simulink model "phasor08_ieee13_2_sc_console"  (Simulink 10.2)
settings: Solver=ode4  StartTime=0.0  StopTime=inf  FixedStep=0.01  RelTol=1e-3
PreLoadFcn:
  | Ts=0.01;
PostLoadFcn:
  | Ts=0.01;
InitFcn:
  | Ts=0.01;
StartFcn:
  | Ts=0.01;
libraries: opal_lib x2
settings Model: Creator=ZhiqiZhao  LastModifiedBy=xjk374
settings DataIOCC: LimitDataPoints=on
settings OptimizationCC: ExpressionDepthLimit=2147483647  LocalBlockOutputs=off
settings DebuggingCC: SolverPrmCheckMsg=warning  AllowSymbolicDim=off  StateNameClashWarn=warning
settings RTWCC: GenCodeOnly=on

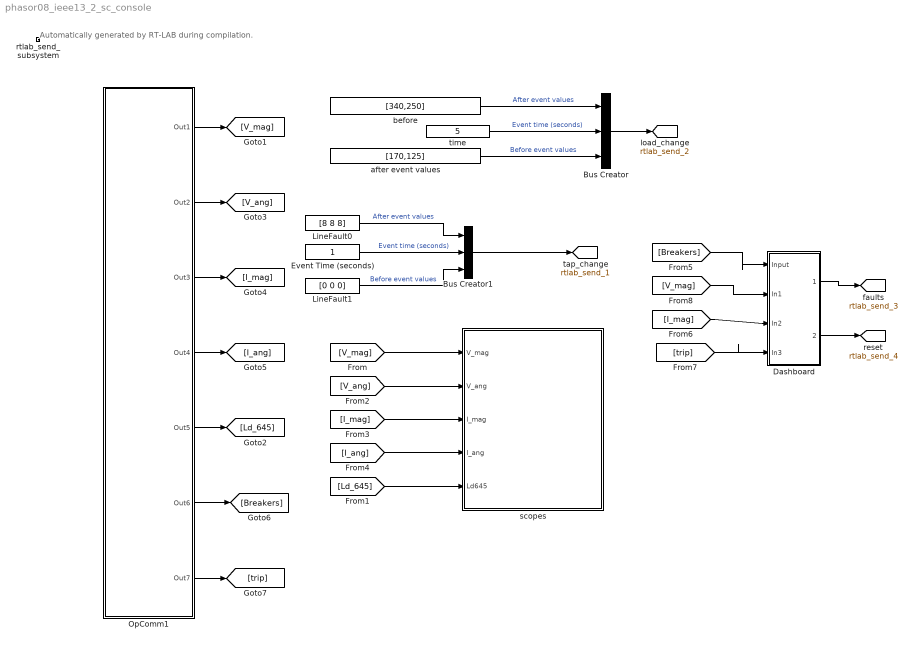
== system phasor08_ieee13_2_sc_console ==
  note: Automatically generated by RT-LAB during compilation.
  Bus Creator : BusCreator  Inputs=3
  Bus Creator1 : BusCreator  Inputs=3
  Dashboard : Subsystem
  Event Time (seconds) : Constant
  LineFault0 : Constant  Value=[8 8 8]
  LineFault1 : Constant  Value=[0 0 0]
  OpComm1 : Subsystem
      mask init:
      | opmaskdisplay('maskdisplay_block',gcb,'disp(''OpComm'')');
      mask Display:
      | patch([0 0.5 0.7 0],[1 1 0 0],[0.7 0.75 0.9]);
      | patch([1 0.53 0.73 1],[1 1 0 0],[1 0.8 0.7]);
      | plot([0 0 1 1 0],[0 1 1 0 0]);
      | disp('OpComm')
  after event values : Constant  Value=[170,125]
  before : Constant  Value=[340,250]
  rtlab_send_subsystem : Subsystem  Priority=-100
      mask Display: text(0,0,'');
  scopes : Subsystem
  time : Constant  Value=5
  tag scope: rtlab_send_1=global, rtlab_send_2=global, rtlab_send_3=global, rtlab_send_4=global
  wires:
  [V_mag] -> Dashboard/2(In1)
  Dashboard/2(Output1) -> [rtlab_send_4]
  [trip] -> Dashboard/4(In3)
  OpComm1/7(Out7) -> [trip]
  [I_mag] -> Dashboard/3(In2)
  Dashboard/1(Output) -> [rtlab_send_3]
  [Breakers] -> Dashboard/1(Input)
  OpComm1/6(Out6) -> [Breakers]
  [Ld_645] -> scopes/5(Ld645)
  [I_ang] -> scopes/4(I_ang)
  [I_mag] -> scopes/3(I_mag)
  [V_ang] -> scopes/2(V_ang)
  [V_mag] -> scopes/1(V_mag)
  OpComm1/3(Out3) -> [I_mag]
  OpComm1/4(Out4) -> [I_ang]
  OpComm1/5(Out5) -> [Ld_645]
  after event values/1 -> Bus Creator/3  "Before event values"
  before/1 -> Bus Creator/1  "After event values"
  Bus Creator1/1 -> [rtlab_send_1]
  Event Time (seconds)/1 -> Bus Creator1/2  "Event time (seconds)"
  LineFault1/1 -> Bus Creator1/3  "Before event values"
  LineFault0/1 -> Bus Creator1/1  "After event values"
  Bus Creator/1 -> [rtlab_send_2]
  time/1 -> Bus Creator/2  "Event time (seconds)"
  OpComm1/2(Out2) -> [V_ang]
  OpComm1/1(Out1) -> [V_mag]

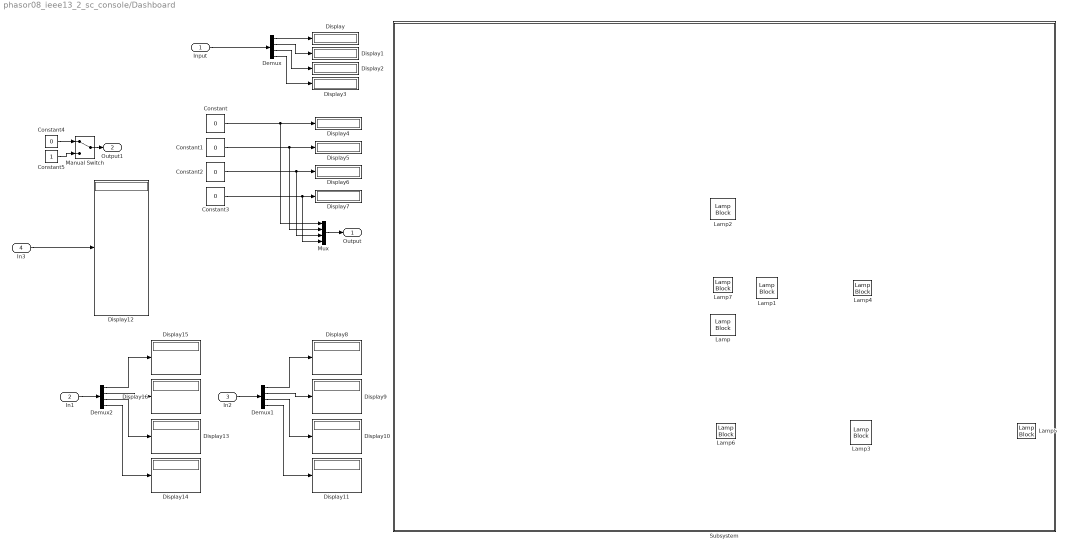
== system phasor08_ieee13_2_sc_console/Dashboard ==
  Input : Inport
  In1 : Inport  Port=2
  In2 : Inport  Port=3
  In3 : Inport  Port=4
  Constant{,1..4} (5 alike) : Constant  Value=0
  Constant5 : Constant
  Demux : Demux
  Demux1 : Demux
  Demux2 : Demux
  Display{,1..16} (17 alike) : Display
  Lamp : LampBlock  LabelPosition=Hide  DefaultColor=DataTag1  States=DataTag2
  Lamp1 : LampBlock  LabelPosition=Hide  DefaultColor=DataTag4  States=DataTag5
  Lamp2 : LampBlock  LabelPosition=Hide  DefaultColor=DataTag7  States=DataTag8
  Lamp3 : LampBlock  LabelPosition=Hide  DefaultColor=DataTag10  States=DataTag11
  Lamp4 : LampBlock  LabelPosition=Hide  DefaultColor=DataTag13  States=DataTag14
  Lamp5 : LampBlock  LabelPosition=Hide  DefaultColor=DataTag16  States=DataTag17
  Lamp6 : LampBlock  LabelPosition=Hide  DefaultColor=DataTag19  States=DataTag20
  Lamp7 : LampBlock  LabelPosition=Hide  DefaultColor=DataTag22  States=DataTag23
  Manual Switch : ManualSwitch
  Mux : Mux
  Subsystem : Subsystem
      mask Display: image('C:\Users\xjk374\OneDrive\0x_Adaptive_Protection\ieee13 with relays.png'); % Use "Edit Image" on toolstrip to change.
  Output : Outport
  Output1 : Outport  Port=2
  wires:
  Demux/1 -> Display/1
  Demux/2 -> Display1/1
  Demux/3 -> Display2/1
  Demux/4 -> Display3/1
  Input/1 -> Demux/1
  Constant/1 -> Mux/1, Display4/1
  Constant1/1 -> Mux/2, Display5/1
  Constant2/1 -> Mux/3, Display6/1
  Constant3/1 -> Mux/4, Display7/1
  Mux/1 -> Output/1
  In2/1 -> Demux1/1
  Demux1/3 -> Display10/1
  Demux1/4 -> Display11/1
  Demux1/2 -> Display9/1
  Demux1/1 -> Display8/1
  In3/1 -> Display12/1
  Constant4/1 -> Manual Switch/1
  Constant5/1 -> Manual Switch/2
  Manual Switch/1 -> Output1/1
  Demux2/1 -> Display15/1
  Demux2/2 -> Display16/1
  Demux2/4 -> Display14/1
  Demux2/3 -> Display13/1
  In1/1 -> Demux2/1

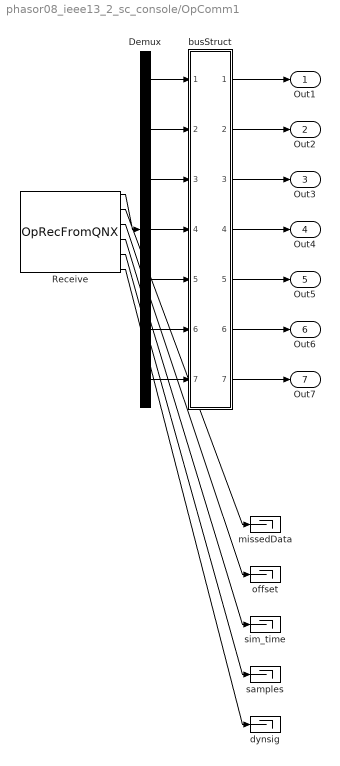
== system phasor08_ieee13_2_sc_console/OpComm1 ==
  Demux : Demux  Outputs="[12  12  12  12   2   4  12]"
  Receive : opal_lib/Communication/OpRecFromQNX  Node_num=1  Acqu_Group=1  Data_Width=66  Synchronization=on  Interpolation=on  Threshold=1.0  modelname=phasor08_IEEE13.mdl  sampletime=0.01
  busStruct : Subsystem
  dynsig : Terminator
  missedData : Terminator
  offset : Terminator
  samples : Terminator
  sim_time : Terminator
  Out1 : Outport
  Out2 : Outport  Port=2
  Out3 : Outport  Port=3
  Out4 : Outport  Port=4
  Out5 : Outport  Port=5
  Out6 : Outport  Port=6
  Out7 : Outport  Port=7
  wires:
  Demux/7 -> busStruct/7(In7)
  Demux/6 -> busStruct/6(In6)
  Demux/5 -> busStruct/5(In5)
  Demux/4 -> busStruct/4(In4)
  Demux/3 -> busStruct/3(In3)
  Demux/2 -> busStruct/2(In2)
  Demux/1 -> busStruct/1(In1)
  busStruct/7(Out7) -> Out7/1
  busStruct/6(Out6) -> Out6/1
  busStruct/5(Out5) -> Out5/1
  busStruct/4(Out4) -> Out4/1
  busStruct/3(Out3) -> Out3/1
  busStruct/2(Out2) -> Out2/1
  busStruct/1(Out1) -> Out1/1
  Receive/1 -> Demux/1
  Receive/6 -> dynsig/1
  Receive/5 -> samples/1
  Receive/4 -> sim_time/1
  Receive/3 -> offset/1
  Receive/2 -> missedData/1

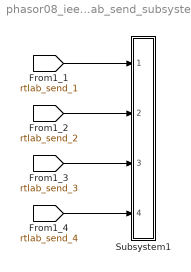
== system phasor08_ieee13_2_sc_console/rtlab_send_subsystem ==
  Subsystem1 : Subsystem
  wires:
  [rtlab_send_1] -> Subsystem1/1(In1)
  [rtlab_send_2] -> Subsystem1/2(In2)
  [rtlab_send_3] -> Subsystem1/3(In3)
  [rtlab_send_4] -> Subsystem1/4(In4)

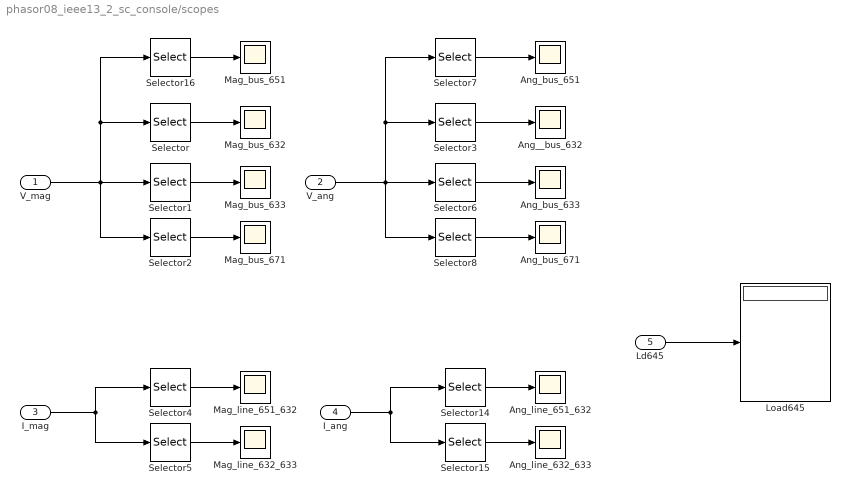
== system phasor08_ieee13_2_sc_console/scopes ==
  V_mag : Inport
  V_ang : Inport  Port=2
  I_mag : Inport  Port=3
  I_ang : Inport  Port=4
  Ld645 : Inport  Port=5
  Ang__bus_632 : Scope
  Ang_bus_633 : Scope
  Ang_bus_651 : Scope
  Ang_bus_671 : Scope
  Ang_line_632_633 : Scope
  Ang_line_651_632 : Scope
  Load645 : Display
  Mag_bus_{632..633,651,671} (4 alike) : Scope
  Mag_line_632_633 : Scope
  Mag_line_651_632 : Scope
  Selector{,3,5,15} (4 alike) : Selector  InputPortWidth=12  IndexOptions=Index vector (dialog)  Indices=[4 5 6]  OutputSizes=1
  Selector1 : Selector  InputPortWidth=12  IndexOptions=Index vector (dialog)  Indices=[7 8 9]  OutputSizes=1
  Selector{4,7,14,16} (4 alike) : Selector  InputPortWidth=12  IndexOptions=Index vector (dialog)  Indices=[1 2 3]  OutputSizes=1
  Selector2 : Selector  InputPortWidth=12  IndexOptions=Index vector (dialog)  Indices=[10 11 12]  OutputSizes=1
  Selector6 : Selector  InputPortWidth=12  IndexOptions=Index vector (dialog)  Indices=[7 8 9]  OutputSizes=1
  Selector8 : Selector  InputPortWidth=12  IndexOptions=Index vector (dialog)  Indices=[10 11 12]  OutputSizes=1
  wires:
  Selector/1 -> Mag_bus_632/1
  Selector1/1 -> Mag_bus_633/1
  Selector2/1 -> Mag_bus_671/1
  V_mag/1 -> Selector1/1, Selector2/1, Selector/1, Selector16/1
  Ld645/1 -> Load645/1
  Selector4/1 -> Mag_line_651_632/1
  Selector14/1 -> Ang_line_651_632/1
  I_ang/1 -> Selector14/1, Selector15/1
  Selector16/1 -> Mag_bus_651/1
  I_mag/1 -> Selector5/1, Selector4/1
  Selector5/1 -> Mag_line_632_633/1
  Selector15/1 -> Ang_line_632_633/1
  V_ang/1 -> Selector8/1, Selector6/1, Selector7/1, Selector3/1
  Selector7/1 -> Ang_bus_651/1
  Selector3/1 -> Ang__bus_632/1
  Selector6/1 -> Ang_bus_633/1
  Selector8/1 -> Ang_bus_671/1

== system phasor08_ieee13_2_sc_console/Dashboard/Subsystem ==

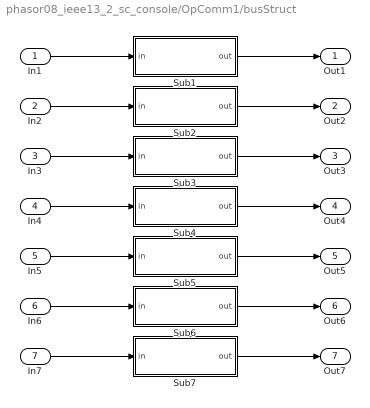
== system phasor08_ieee13_2_sc_console/OpComm1/busStruct ==
  In1 : Inport
  In2 : Inport  Port=2
  In3 : Inport  Port=3
  In4 : Inport  Port=4
  In5 : Inport  Port=5
  In6 : Inport  Port=6
  In7 : Inport  Port=7
  Sub1 : Subsystem
  Sub2 : Subsystem
  Sub3 : Subsystem
  Sub4 : Subsystem
  Sub5 : Subsystem
  Sub6 : Subsystem
  Sub7 : Subsystem
  Out1 : Outport
  Out2 : Outport  Port=2
  Out3 : Outport  Port=3
  Out4 : Outport  Port=4
  Out5 : Outport  Port=5
  Out6 : Outport  Port=6
  Out7 : Outport  Port=7
  wires:
  Sub7/1(out) -> Out7/1
  In7/1 -> Sub7/1(in)
  Sub6/1(out) -> Out6/1
  In6/1 -> Sub6/1(in)
  Sub5/1(out) -> Out5/1
  In5/1 -> Sub5/1(in)
  Sub4/1(out) -> Out4/1
  In4/1 -> Sub4/1(in)
  Sub3/1(out) -> Out3/1
  In3/1 -> Sub3/1(in)
  Sub2/1(out) -> Out2/1
  In2/1 -> Sub2/1(in)
  Sub1/1(out) -> Out1/1
  In1/1 -> Sub1/1(in)

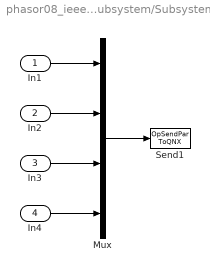
== system phasor08_ieee13_2_sc_console/rtlab_send_subsystem/Subsystem1 ==
  In1 : Inport  PortDimensions=7
  In2 : Inport  Port=2  PortDimensions=5
  In3 : Inport  Port=3  PortDimensions=4
  In4 : Inport  Port=4  PortDimensions=1
  Mux : Mux
  Send1 : opal_lib/Communication/OpSendPar ToQNX  Node_num=1  modelname=phasor08_IEEE13
  wires:
  Mux/1 -> Send1/1
  In1/1 -> Mux/1
  In2/1 -> Mux/2
  In3/1 -> Mux/3
  In4/1 -> Mux/4

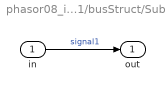
== system phasor08_ieee13_2_sc_console/OpComm1/busStruct/Sub1 ==
  in : Inport
  out : Outport
  wires:
  in/1 -> out/1  "signal1"

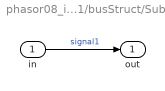
== system phasor08_ieee13_2_sc_console/OpComm1/busStruct/Sub2 ==
  in : Inport
  out : Outport
  wires:
  in/1 -> out/1  "signal1"

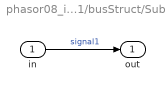
== system phasor08_ieee13_2_sc_console/OpComm1/busStruct/Sub3 ==
  in : Inport
  out : Outport
  wires:
  in/1 -> out/1  "signal1"

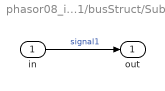
== system phasor08_ieee13_2_sc_console/OpComm1/busStruct/Sub4 ==
  in : Inport
  out : Outport
  wires:
  in/1 -> out/1  "signal1"

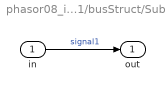
== system phasor08_ieee13_2_sc_console/OpComm1/busStruct/Sub5 ==
  in : Inport
  out : Outport
  wires:
  in/1 -> out/1  "signal1"

== system phasor08_ieee13_2_sc_console/OpComm1/busStruct/Sub6 ==
  in : Inport
  out : Outport
  wires:
  in/1 -> out/1  "signal1"

== system phasor08_ieee13_2_sc_console/OpComm1/busStruct/Sub7 ==
  in : Inport
  out : Outport
  wires:
  in/1 -> out/1  "signal1"
